simulink model "model1"  (R2020b)
settings: Solver=VariableStepAuto  StartTime=0.0  StopTime=50  MaxStep=1e-5  RelTol=1e-3
settings Model: Creator=lulut  LastModifiedBy=lulut
settings SolverCC: MaxConsecutiveMinStep=3  ZeroCrossControl=EnableAll  ZeroCrossAlgorithm=Adaptive

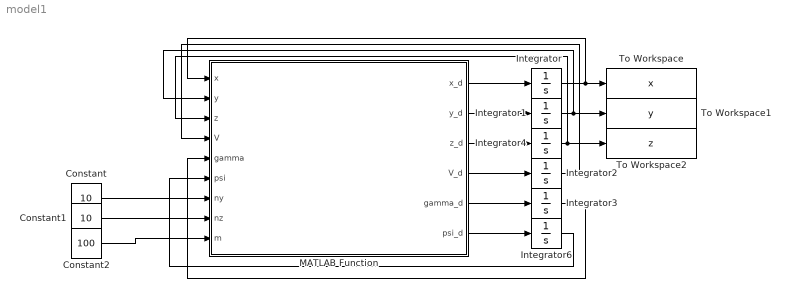
== system model1 ==
  Constant : Constant  Value=10
  Constant1 : Constant  Value=10
  Constant2 : Constant  Value=100
  Integrator{,1,3,6} (4 alike) : Integrator
  Integrator2 : Integrator  InitialCondition=280
  Integrator4 : Integrator  InitialCondition=300
  MATLAB Function : MATLAB Function  TreatAsAtomicUnit=on
  To Workspace : ToWorkspace  VariableName=x  SampleTime=-1
  To Workspace1 : ToWorkspace  VariableName=y  SampleTime=-1
  To Workspace2 : ToWorkspace  VariableName=z  SampleTime=-1
  wires:
  MATLAB Function/1(x_d) -> Integrator/1
  MATLAB Function/2(y_d) -> Integrator1/1
  MATLAB Function/3(z_d) -> Integrator4/1
  MATLAB Function/4(V_d) -> Integrator2/1
  MATLAB Function/5(gamma_d) -> Integrator3/1
  MATLAB Function/6(psi_d) -> Integrator6/1
  Integrator/1 -> To Workspace/1, MATLAB Function/1(x)
  Integrator1/1 -> To Workspace1/1, MATLAB Function/2(y)
  Integrator4/1 -> To Workspace2/1, MATLAB Function/3(z)
  Integrator2/1 -> MATLAB Function/4(V)
  Integrator3/1 -> MATLAB Function/5(gamma)
  Integrator6/1 -> MATLAB Function/6(psi)
  Constant/1 -> MATLAB Function/7(ny)
  Constant1/1 -> MATLAB Function/8(nz)
  Constant2/1 -> MATLAB Function/9(m)

== matlab function model1/MATLAB Function ==
  data: x input double size=1; x_d output double size=1; y input double size=1; z input double size=1; V input double size=1; gamma input double size=1; psi input double size=1; ny input double size=1; nz input double size=1; m input double size=1; y_d output double size=1; z_d output double size=1; V_d output double size=1; gamma_d output double size=1; psi_d output double size=1
function [x_d,y_d,z_d,V_d,gamma_d,psi_d] = model_1(x, y, z ,V, gamma ,psi,ny,nz,m)

%这是主要考虑过载控制的仿真模型
%ny和nz表示垂直于速度方向的两个过载，为动力学模型的控制输入
%status = [x y z V gamma psi]
S_ref = 1; %飞行器特征面积
C_d = 0.25; %飞行器阻力系数
g = 9.8061;  %平面大地假设下的重力加速度
rou_0 = 1.225; %海平面空气密度
H = 7200;  %大气密度计算常值

rou = rou_0 * exp(-z/H);
D = 0.5 * rou * V^2 * S_ref * C_d;
x_d = V * cos(gamma) * sin(psi);
y_d = V * cos(gamma) * cos(psi);
z_d = V * sin(gamma);
V_d = -D/m - g*sin(gamma);
gamma_d = ny/V;
psi_d = nz/(V * cos(gamma));
